simulink model "closedloop_1D"  (R2016b)
settings: Solver=VariableStepAuto  StartTime=0.0  StopTime=10.0  FixedStep=0.0001  RelTol=1e-3
values from neighbouring files (symbols this model uses):
  g = 9.81    [NL_1D_Model.m]
  I_GO = I_KO+I_RM+m_r*l_M^2    (= 0.00355187)    [NL_1D_Model.m]
  I_RM = 1.1683e-4    (= 0.00011683)    [NL_1D_Model.m]
  k = [-0.9120, -0.0773, -0.0001]    [NL_1D_Model.m]
  l_C = (l_M*m_r+l_AC*m_k)/m_g    [NL_1D_Model.m]    (also in NL_3D_Model.m = 0.066)
  m = m_r + m_k    (= 0.311)    [NL_1D_Model.m]    (also in NL_3D_Model.m = 1.532)
  u_max = 0.07    [NL_1D_Model.m]
  x_0 = degtorad([3;0;0])    [NL_1D_Model.m]    (also in NL_3D_Model_u_limited.m = [x_0;zeros(6,1)]; NL_3D_Model_u_limited_x_offset.m = [x_0;zeros(6,1)])
settings Model: Creator=michael  LastModifiedBy=michael

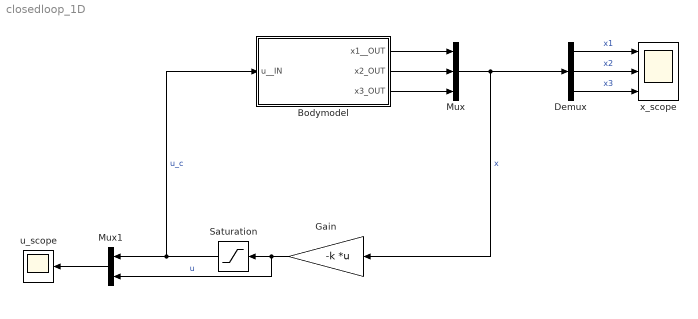
== system closedloop_1D ==
  Bodymodel : Subsystem
  Demux : Demux  Outputs=3
  Gain : Gain  Gain=-k  Multiplication=Matrix(K*u)
  Mux : Mux  Inputs=3
  Mux1 : Mux  Inputs=2
  Saturation : Saturate  UpperLimit=u_max  LowerLimit=-u_max
  u_scope : Scope
  x_scope : Scope  NumInputPorts=3
  wires:
  Gain/1 -> Mux1/2, Saturation/1  "u"
  Bodymodel/2(x2_OUT) -> Mux/2
  Bodymodel/1(x1__OUT) -> Mux/1
  Bodymodel/3(x3_OUT) -> Mux/3
  Mux/1 -> Demux/1, Gain/1  "x"
  Demux/1 -> x_scope/1  "x1"
  Demux/2 -> x_scope/2  "x2"
  Demux/3 -> x_scope/3  "x3"
  Saturation/1 -> Mux1/1, Bodymodel/1(u__IN)  "u_c"
  Mux1/1 -> u_scope/1

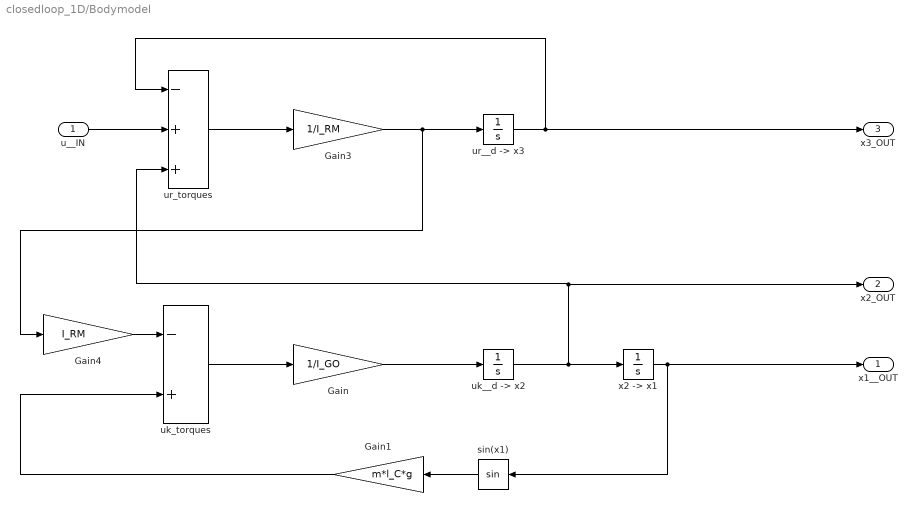
== system closedloop_1D/Bodymodel ==
  u__IN : Inport
  Gain : Gain  Gain=1/I_GO
  Gain1 : Gain  Gain=m*l_C*g
  Gain3 : Gain  Gain=1/I_RM
  Gain4 : Gain  Gain=I_RM
  sin(x1) : Trigonometry
  "uk__d -> x2" : Integrator  InitialCondition=x_0(2)
  uk_torques : Sum  Inputs=-+
  "ur__d -> x3" : Integrator  InitialCondition=x_0(3)
  ur_torques : Sum  Inputs=-++
  "x2 -> x1" : Integrator  InitialCondition=x_0(1)
  x1__OUT : Outport
  x2_OUT : Outport  Port=2
  x3_OUT : Outport  Port=3
  wires:
  "uk__d -> x2"/1 -> "x2 -> x1"/1, ur_torques/3, x2_OUT/1
  Gain/1 -> "uk__d -> x2"/1
  uk_torques/1 -> Gain/1
  "x2 -> x1"/1 -> x1__OUT/1, sin(x1)/1
  sin(x1)/1 -> Gain1/1
  Gain1/1 -> uk_torques/2
  "ur__d -> x3"/1 -> x3_OUT/1, ur_torques/1
  ur_torques/1 -> Gain3/1
  u__IN/1 -> ur_torques/2
  Gain3/1 -> Gain4/1, "ur__d -> x3"/1
  Gain4/1 -> uk_torques/1
